simulink model "st_lab6"  (R2025b)
settings: Solver=ode4  StartTime=0.0  StopTime=25  FixedStep=1e-4  RelTol=1e-3
undefined symbols (not defined in the file or in its folder): C, L, R
settings Model: Creator=vladl  LastModifiedBy=vladl

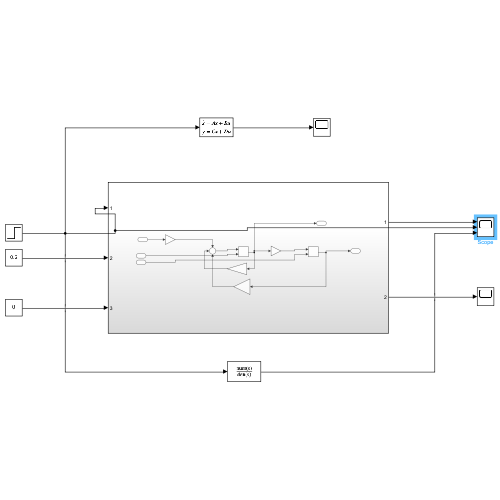
[thumbnail: Simulink's stored preview of the top-level diagram]
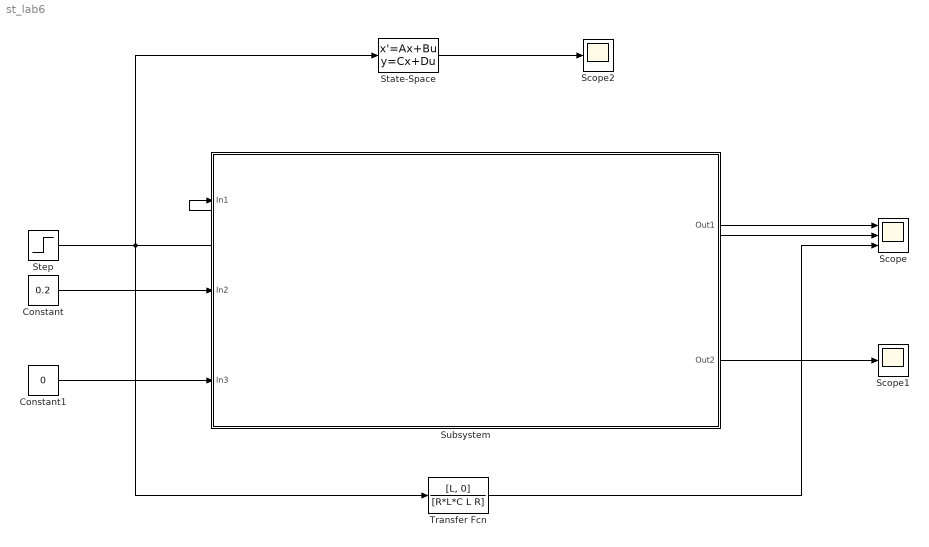
== system st_lab6 ==
  Constant : Constant  Value=0.2
  Constant1 : Constant  Value=0
  Scope : Scope  NumInputPorts=3
      settings: ActiveDisplayYMinimum=-2.3872237409193149  ActiveDisplayYMaximum=5.4884598948608776
  Scope1 : Scope
      settings: ActiveDisplayYMinimum=-0.52457152034141641  ActiveDisplayYMaximum=1.5628215571833484
  Scope2 : Scope
      settings: ActiveDisplayYMinimum=-4.2024392998905311  ActiveDisplayYMaximum=13.239631052188111  DataLoggingVariableName=ScopeData2
  State-Space : StateSpace  A=[-1/(R*C) -1/C; 1/L 0]  B=[1/(R*C); 0]  C=[1 0]  D=0  InitialCondition=0
  Step : Step  After=10  SampleTime=0
  Subsystem : Subsystem
  Transfer Fcn : TransferFcn  Numerator=[L, 0]  Denominator=[R*L*C L R]
  wires:
  Step/1 -> Transfer Fcn/1, State-Space/1, Subsystem/1(In1), Scope/2
  Subsystem/1(Out1) -> Scope/1
  Subsystem/2(Out2) -> Scope1/1
  Constant/1 -> Subsystem/2(In2)
  Constant1/1 -> Subsystem/3(In3)
  State-Space/1 -> Scope2/1
  Transfer Fcn/1 -> Scope/3

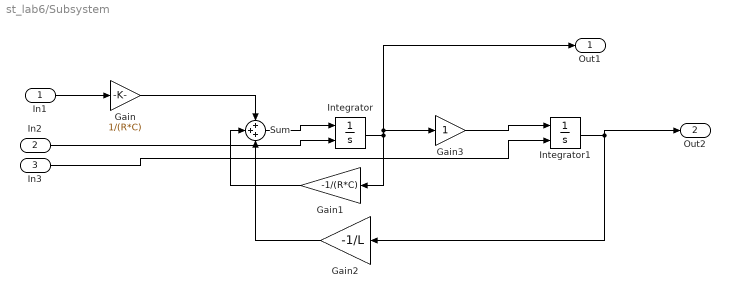
== system st_lab6/Subsystem ==
  In1 : Inport
  In2 : Inport  Port=2
  In3 : Inport  Port=3
  Gain : Gain  Gain=1/(R*C)
  Gain1 : Gain  Gain=-1/(R*C)
  Gain2 : Gain  Gain=-1/L
  Gain3 : Gain
  Integrator : Integrator  InitialConditionSource=external
  Integrator1 : Integrator  InitialConditionSource=external
  Sum : Sum  Inputs=+++
  Out1 : Outport
  Out2 : Outport  Port=2
  wires:
  Gain3/1 -> Integrator1/1
  Integrator/1 -> Out1/1, Gain3/1, Gain1/1
  Gain2/1 -> Sum/3
  In1/1 -> Gain/1
  Integrator1/1 -> Out2/1, Gain2/1
  Sum/1 -> Integrator/1
  Gain1/1 -> Sum/2
  Gain/1 -> Sum/1
  In2/1 -> Integrator/2
  In3/1 -> Integrator1/2
